simulink model "Automated_features1"  (R2020b)
settings: Solver=VariableStepAuto  StartTime=0.0  StopTime=10.0  RelTol=1e-3
undefined symbols (not defined in the file): sigbuilder_block
libraries: simulink x126
(part 1 of 3)
settings Model: Creator=99003762  LastModifiedBy=99003728
settings SFSimCC: CustomCodeUndefinedFunction=UseInterfaceOnly

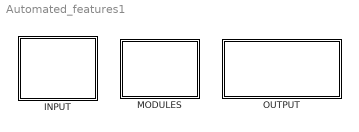
== system Automated_features1 ==
  INPUT : Subsystem
  MODULES : Subsystem
  OUTPUT : Subsystem

== system Automated_features1/INPUT ==
  note: Tier pressure sensors and Roof Control Inputs
  AIRBAG_INPUTS : Subsystem
  ALARM_INPUTS : Subsystem
  Cruise_Control_INPUT : Subsystem
  Power_window_ip : Subsystem  Tag=power_ip
  SEAT_RESTRAINT_INPUTS : Subsystem
  Signal Builder : Subsystem  Tag=STV Subsys  LoadFcn=sigbuilder_block('load');  StartFcn=sigbuilder_block('start');  StopFcn=sigbuilder_block('stop');  ClipboardFcn=sigbuilder_block('clipboard');  mask(Sigbuilder block){tuvar=[0:10]}
      mask help: Simulink:masks:SigbuilderBlock_MD
      mask init:
      | if ~strcmp(get_param(bdroot(gcbh),'SimulationStatus'),'stopped') tuvar = sigbuilder_block('maskInit'); end
      settings: CopyFcn=sigbuilder_block('copy');  DeleteFcn=sigbuilder_block('delete');  ModelCloseFcn=sigbuilder_block('modelClose');  PreSaveFcn=sigbuilder_block('preSave');  PauseFcn=sigbuilder_block('pause');  ContinueFcn=sigbuilder_block('continue');  NameChangeFcn=sigbuilder_block('namechange');  OpenFcn=sigbuilder_block('open',[6 30 1188 546.75 ]);  CloseFcn=sigbuilder_block('close');
      mask Display: plot(0, 0, 100, 100,[2, 2, 32, 32, 2], [68, 8, 8, 68, 68],[32, 2], [38, 38], [32, 19, 2],[53, 60, 44], [32, 17, 17, 2],[16, 16, 31, 31]);txt = getActiveGroup(gcbh);text(2, 100, txt,'verticalAlignment', 'top');
  Wiper_INPUTS : Subsystem
  tag scope: CL_SW=global, CL_VAL=global, OP_SW=global, OP_VAL=global, TP1_IP=global, TP2=global, TP3=global, TP4=global
  wires:
  Signal Builder/2(TP2) -> [TP2]
  Signal Builder/7(OPEN_VALUE) -> [OP_VAL]
  Signal Builder/1(TP1) -> [TP1_IP]
  Signal Builder/6(CLOSE_SW) -> [CL_SW]
  Signal Builder/4(TP4) -> [TP4]
  Signal Builder/3(TP3) -> [TP3]
  Signal Builder/5(OPEN_SW) -> [OP_SW]
  Signal Builder/8(CLOSE_VALUE) -> [CL_VAL]

== system Automated_features1/MODULES ==
  "\tPOWER_WINDOW" : Subsystem
  AIRBAGSYSTEM : Subsystem
  ALARM_SYSTEM : Subsystem
  CRUISE_CONTROL : Subsystem
  SeatBelt_MODULE : Subsystem
  Tire Pressure Monitoring System : Subsystem
  WIPER_CONTROL : Subsystem
  sunroof : Subsystem
  tag scope: CushionAngle=global, FrontAngle=global, RearAngle=global, SeatAdj=global
  wires:
  SeatBelt_MODULE/4(CushionAdjustAngle) -> [CushionAngle]
  SeatBelt_MODULE/2(RearAdjustAngle) -> [RearAngle]
  SeatBelt_MODULE/3(SeatAdjust) -> [SeatAdj]
  SeatBelt_MODULE/1(FrontAdjustAngle) -> [FrontAngle]

== system Automated_features1/OUTPUT ==
  note: sunroof Display
  note: Tyre pressure Indicators
  AIRBAG_OUTPUTS : Subsystem
  ALARM_OUTPUT1 : Subsystem
  Cruise_output : Subsystem
  OUTPUT1 : Subsystem
  OUTPUT2 : Subsystem
  Power_window_OUTPUT : Subsystem
  SeatBelt_OUTPUTS : Subsystem
  TP1_Indicator : LampBlock
  TP2_Indicator : LampBlock
  TP3_Indicator : LampBlock
  TP4_Indicator : LampBlock

== system Automated_features1/INPUT/AIRBAG_INPUTS ==
  Signal Builder : Subsystem  Tag=STV Subsys  LoadFcn=sigbuilder_block('load');  StartFcn=sigbuilder_block('start');  StopFcn=sigbuilder_block('stop');  ClipboardFcn=sigbuilder_block('clipboard');  mask(Sigbuilder block){tuvar=[0:10]}
      mask help: Simulink:masks:SigbuilderBlock_MD
      mask init:
      | if ~strcmp(get_param(bdroot(gcbh),'SimulationStatus'),'stopped') tuvar = sigbuilder_block('maskInit'); end
      settings: CopyFcn=sigbuilder_block('copy');  DeleteFcn=sigbuilder_block('delete');  ModelCloseFcn=sigbuilder_block('modelClose');  PreSaveFcn=sigbuilder_block('preSave');  PauseFcn=sigbuilder_block('pause');  ContinueFcn=sigbuilder_block('continue');  NameChangeFcn=sigbuilder_block('namechange');  OpenFcn=sigbuilder_block('open',[437.6 199.2 550.4 400 ]);  CloseFcn=sigbuilder_block('close');
      mask Display: plot(0, 0, 100, 100,[2, 2, 32, 32, 2], [68, 8, 8, 68, 68],[32, 2], [38, 38], [32, 19, 2],[53, 60, 44], [32, 17, 17, 2],[16, 16, 31, 31]);txt = getActiveGroup(gcbh);text(2, 100, txt,'verticalAlignment', 'top');
  tag scope: Air_ACC=global, Driver_L=global, L_Front_1=global, L_Rear_1=global, R_Rear_=global, VehicleSpeed=global, YawRate=global
  wires:
  Signal Builder/1(Driver_L) -> [Driver_L]
  Signal Builder/2(L_Front_1) -> [L_Front_1]
  Signal Builder/3(L_Rear_1) -> [L_Rear_1]
  Signal Builder/4(R_Rear_) -> [R_Rear_]
  Signal Builder/5(VehicleSpeed) -> [VehicleSpeed]
  Signal Builder/6(Air_ACC) -> [Air_ACC]
  Signal Builder/7(YawRate) -> [YawRate]

== system Automated_features1/INPUT/ALARM_INPUTS ==
  Signal Builder : Subsystem  Tag=STV Subsys  LoadFcn=sigbuilder_block('load');  StartFcn=sigbuilder_block('start');  StopFcn=sigbuilder_block('stop');  ClipboardFcn=sigbuilder_block('clipboard');  mask(Sigbuilder block){tuvar=[0:10]}
      mask help: Simulink:masks:SigbuilderBlock_MD
      mask init:
      | if ~strcmp(get_param(bdroot(gcbh),'SimulationStatus'),'stopped') tuvar = sigbuilder_block('maskInit'); end
      settings: CopyFcn=sigbuilder_block('copy');  DeleteFcn=sigbuilder_block('delete');  ModelCloseFcn=sigbuilder_block('modelClose');  PreSaveFcn=sigbuilder_block('preSave');  PauseFcn=sigbuilder_block('pause');  ContinueFcn=sigbuilder_block('continue');  NameChangeFcn=sigbuilder_block('namechange');  OpenFcn=sigbuilder_block('open',[403.5 199.2 550.5 359.55 ]);  CloseFcn=sigbuilder_block('close');
      mask Display: plot(0, 0, 100, 100,[2, 2, 32, 32, 2], [68, 8, 8, 68, 68],[32, 2], [38, 38], [32, 19, 2],[53, 60, 44], [32, 17, 17, 2],[16, 16, 31, 31]);txt = getActiveGroup(gcbh);text(2, 100, txt,'verticalAlignment', 'top');
  tag scope: AS_Doors=global, CAR_ON=global, Ignition=global, RKE=global
  wires:
  Signal Builder/1(AS_Doors) -> [AS_Doors]
  Signal Builder/2(Ignition) -> [Ignition]
  Signal Builder/3(Car_ON) -> [CAR_ON]
  Signal Builder/4(RKE) -> [RKE]

== system Automated_features1/INPUT/Cruise_Control_INPUT ==
  Signal Builder : Subsystem  Tag=STV Subsys  LoadFcn=sigbuilder_block('load');  StartFcn=sigbuilder_block('start');  StopFcn=sigbuilder_block('stop');  ClipboardFcn=sigbuilder_block('clipboard');  mask(Sigbuilder block){tuvar=[0:10]}
      mask help: Simulink:masks:SigbuilderBlock_MD
      mask init:
      | if ~strcmp(get_param(bdroot(gcbh),'SimulationStatus'),'stopped') tuvar = sigbuilder_block('maskInit'); end
      settings: CopyFcn=sigbuilder_block('copy');  DeleteFcn=sigbuilder_block('delete');  ModelCloseFcn=sigbuilder_block('modelClose');  PreSaveFcn=sigbuilder_block('preSave');  PauseFcn=sigbuilder_block('pause');  ContinueFcn=sigbuilder_block('continue');  NameChangeFcn=sigbuilder_block('namechange');  OpenFcn=sigbuilder_block('open',[437.6 153 550.4 359.25 ]);  CloseFcn=sigbuilder_block('close');
      mask Display: plot(0, 0, 100, 100,[2, 2, 32, 32, 2], [68, 8, 8, 68, 68],[32, 2], [38, 38], [32, 19, 2],[53, 60, 44], [32, 17, 17, 2],[16, 16, 31, 31]);txt = getActiveGroup(gcbh);text(2, 100, txt,'verticalAlignment', 'top');
  tag scope: BRAKE_CC=global, CRUISE_SPEED_CHANGE_SW=global, CRUISE_SWITCH=global, DESIRED_SPEED_CRUISE=global, ESC_cc=global, IGN=global, SPEED_CONTROL_CC=global, TSC_CC=global
  wires:
  Signal Builder/4(Ignition) -> [IGN]  "igswitch"
  Signal Builder/6(Cruise_switch) -> [CRUISE_SWITCH]
  Signal Builder/3(BRAKE) -> [BRAKE_CC]
  Signal Builder/5(desired_speed) -> [DESIRED_SPEED_CRUISE]
  Signal Builder/7(Speed_enable) -> [CRUISE_SPEED_CHANGE_SW]
  Signal Builder/2(TSC) -> [TSC_CC]
  Signal Builder/1(ESC) -> [ESC_cc]
  Signal Builder/8(Cruise_speed_change_sw) -> [SPEED_CONTROL_CC]

== system Automated_features1/INPUT/Power_window_ip ==
  Signal Builder : Subsystem  Tag=STV Subsys  LoadFcn=sigbuilder_block('load');  StartFcn=sigbuilder_block('start');  StopFcn=sigbuilder_block('stop');  ClipboardFcn=sigbuilder_block('clipboard');  mask(Sigbuilder block){tuvar=[0:10]}
      mask help: Simulink:masks:SigbuilderBlock_MD
      mask init:
      | if ~strcmp(get_param(bdroot(gcbh),'SimulationStatus'),'stopped') tuvar = sigbuilder_block('maskInit'); end
      settings: CopyFcn=sigbuilder_block('copy');  DeleteFcn=sigbuilder_block('delete');  ModelCloseFcn=sigbuilder_block('modelClose');  PreSaveFcn=sigbuilder_block('preSave');  PauseFcn=sigbuilder_block('pause');  ContinueFcn=sigbuilder_block('continue');  NameChangeFcn=sigbuilder_block('namechange');  OpenFcn=sigbuilder_block('open',[6 6 1012.5 506.25 ]);  CloseFcn=sigbuilder_block('close');
      mask Display: plot(0, 0, 100, 100,[2, 2, 32, 32, 2], [68, 8, 8, 68, 68],[32, 2], [38, 38], [32, 19, 2],[53, 60, 44], [32, 17, 17, 2],[16, 16, 31, 31]);txt = getActiveGroup(gcbh);text(2, 100, txt,'verticalAlignment', 'top');
  tag scope: Front_left_button_CP=global, Front_left_button_driver_side=global, driver_switch=global, ignition=global, lock_unlock_button=global, object=global, rear_left_button_CP=global, rear_left_button_driver_side=global, rear_right_button_CP=global, rear_right_button_driver_side=global
  wires:
  Signal Builder/5(Front_left_DC) -> [Front_left_button_driver_side]
  Signal Builder/9(Lock_Unlock) -> [lock_unlock_button]
  Signal Builder/6(rear_left_DC) -> [rear_left_button_driver_side]
  Signal Builder/8(oject_detection) -> [object]
  Signal Builder/3(Right_right_CP) -> [rear_right_button_CP]
  Signal Builder/7(rear_right_DC) -> [rear_right_button_driver_side]
  Signal Builder/2(Right_left_CP) -> [rear_left_button_CP]
  Signal Builder/1(Front_left_CP) -> [Front_left_button_CP]
  Signal Builder/10(iginition) -> [ignition]
  Signal Builder/4(Driver_control) -> [driver_switch]

== system Automated_features1/INPUT/SEAT_RESTRAINT_INPUTS ==
  tag scope: AdjustCushionAngle=global, AdjustFrontSeatAngle=global, AdjustRearSeatAngle=global, AdjustSeat=global, FrontSeat=global, HandleOn=global, ModeSelection=global, PowerSeat=global

== system Automated_features1/INPUT/Signal Builder ==
  Demux : Demux  Tag=STV Demux  Outputs=8
      settings: DisplayOption=none
  FromWs : FromWorkspace  Tag=STV FromWs  VariableName=tuvar  SampleTime=1
      SigBuilderData=|
      | common.afterFinalStr = 'Extrapolate'
      | common.sampleTime = '1'
      | dataSet.timeRange = [0 14]
      | dataSet.name = 'Sheet1'
      | sbobj.Name = 'Signal Builder'
      | sbobj.Groups.Name = 'Sheet1'
      | sbobj.Groups.Signals(1).Name = 'TP1'
      | sbobj.Groups.Signals(1).XData = [0 1 2 3 4 5 6 7 8 9 10 11 12 13 14]
      | sbobj.Groups.Signals(1).YData = [76 40 12 45 30 78 72 80 0 85 99 90 14 77 96]
      | sbobj.Groups.Signals(2).Name = 'TP2'
      | sbobj.Groups.Signals(2).XData = [0 1 2 3 4 5 6 7 8 9 10 11 12 13 14]
      | sbobj.Groups.Signals(2).YData = [76 40 96 45 30 78 72 80 0 85 99 90 14 77 96]
      | sbobj.Groups.Signals(3).Name = 'TP3'
      | sbobj.Groups.Signals(3).XData = [0 1 2 3 4 5 6 7 8 9 10 11 12 13 14]
      | sbobj.Groups.Signals(3).YData = [76 40 12 89 30 78 72 80 0 85 99 90 14 77 96]
      | sbobj.Groups.Signals(4).Name = 'TP4'
      | sbobj.Groups.Signals(4).XData = [0 1 2 3 4 5 6 7 8 9 10 11 12 13 14]
      | sbobj.Groups.Signals(4).YData = [76 80 82 45 1 78 72 80 0 85 99 90 14 77 96]
      | sbobj.Groups.Signals(5).Name = 'OPEN_SW'
      | sbobj.Groups.Signals(5).XData = [0 1 2 3 4 5 6 7 8 9 10 11 12 13 14]
      | sbobj.Groups.Signals(5).YData = [0 0 0 0 0 0 0 0 1 1 1 1 1 1 1]
      | sbobj.Groups.Signals(6).Name = 'CLOSE_SW'
      | sbobj.Groups.Signals(6).XData = [0 1 2 3 4 5 6 7 8 9 10 11 12 13 14]
      | sbobj.Groups.Signals(6).YData = [1 0 1 1 1 1 1 1 1 0 0 0 0 0 0]
      | sbobj.Groups.Signals(7).Name = 'OPEN_VALUE'
      | sbobj.Groups.Signals(7).XData = [0 1 2 3 4 5 6 7 8 9 10 11 12 13 14]
      | sbobj.Groups.Signals(7).YData = [76 40 12 45 30 78 72 80 0 85 99 90 14 77 96]
      | sbobj.Groups.Signals(8).Name = 'CLOSE_VALUE'
      | sbobj.Groups.Signals(8).XData = [0 1 2 3 4 5 6 7 8 9 10 11 12 13 14]
      | sbobj.Groups.Signals(8).YData = [76 40 12 45 30 78 72 80 0 85 99 90 14 77 96]
      | sbobj.Groups.TimeRange = [0 14]
  TP1 : Outport  Tag=STV Outport
  TP2 : Outport  Tag=STV Outport  Port=2
  TP3 : Outport  Tag=STV Outport  Port=3
  TP4 : Outport  Tag=STV Outport  Port=4
  OPEN_SW : Outport  Tag=STV Outport  Port=5
  CLOSE_SW : Outport  Tag=STV Outport  Port=6
  OPEN_VALUE : Outport  Tag=STV Outport  Port=7
  CLOSE_VALUE : Outport  Tag=STV Outport  Port=8
  wires:
  Demux/1 -> TP1/1
  FromWs/1 -> Demux/1
  Demux/2 -> TP2/1
  Demux/3 -> TP3/1
  Demux/4 -> TP4/1
  Demux/5 -> OPEN_SW/1
  Demux/6 -> CLOSE_SW/1
  Demux/7 -> OPEN_VALUE/1
  Demux/8 -> CLOSE_VALUE/1

== system Automated_features1/INPUT/Wiper_INPUTS ==
  Signal Builder : Subsystem  Tag=STV Subsys  LoadFcn=sigbuilder_block('load');  StartFcn=sigbuilder_block('start');  StopFcn=sigbuilder_block('stop');  ClipboardFcn=sigbuilder_block('clipboard');  mask(Sigbuilder block){tuvar=[0:10]}
      mask help: Simulink:masks:SigbuilderBlock_MD
      mask init:
      | if ~strcmp(get_param(bdroot(gcbh),'SimulationStatus'),'stopped') tuvar = sigbuilder_block('maskInit'); end
      settings: CopyFcn=sigbuilder_block('copy');  DeleteFcn=sigbuilder_block('delete');  ModelCloseFcn=sigbuilder_block('modelClose');  PreSaveFcn=sigbuilder_block('preSave');  PauseFcn=sigbuilder_block('pause');  ContinueFcn=sigbuilder_block('continue');  NameChangeFcn=sigbuilder_block('namechange');  OpenFcn=sigbuilder_block('open',[437.6 199.2 550.4 400 ]);  CloseFcn=sigbuilder_block('close');
      mask Display: plot(0, 0, 100, 100,[2, 2, 32, 32, 2], [68, 8, 8, 68, 68],[32, 2], [38, 38], [32, 19, 2],[53, 60, 44], [32, 17, 17, 2],[16, 16, 31, 31]);txt = getActiveGroup(gcbh);text(2, 100, txt,'verticalAlignment', 'top');
  tag scope: FC_ManualInput=global, FW_Modes=global, WC_BackS=global, WC_FrontS=global, WC_Status=global
  wires:
  Signal Builder/1(FC_Modes) -> [FW_Modes]
  Signal Builder/2(FC_ManualInput) -> [FC_ManualInput]
  Signal Builder/3(WC_BackS) -> [WC_BackS]
  Signal Builder/4(WC_Fronts) -> [WC_FrontS]
  Signal Builder/5(WC_Status) -> [WC_Status]

== system Automated_features1/MODULES/	POWER_WINDOW ==
  Subsystem4 : Subsystem
  tag scope: FL_out=global, FL_warn=global, RL_out=global, RL_warn=global, RR_out=global, RR_warn=global, driver_side_output=global, driver_warn=global
  wires:
  Subsystem4/2(Out_FL) -> [FL_out]
  Subsystem4/1(Out_warn) -> [FL_warn]
  Subsystem4/4(Out_RL) -> [RL_out]
  Subsystem4/6(Out_RR) -> [RR_out]
  [object] -> Subsystem4/2(object)
  [ignition] -> Subsystem4/1(Ig_sw)
  Subsystem4/3(Out_RL_warn) -> [RL_warn]
  Subsystem4/8(Out_DC) -> [driver_side_output]
  Subsystem4/5(Out_RR_warn) -> [RR_warn]
  Subsystem4/7(Out_DC_warn) -> [driver_warn]

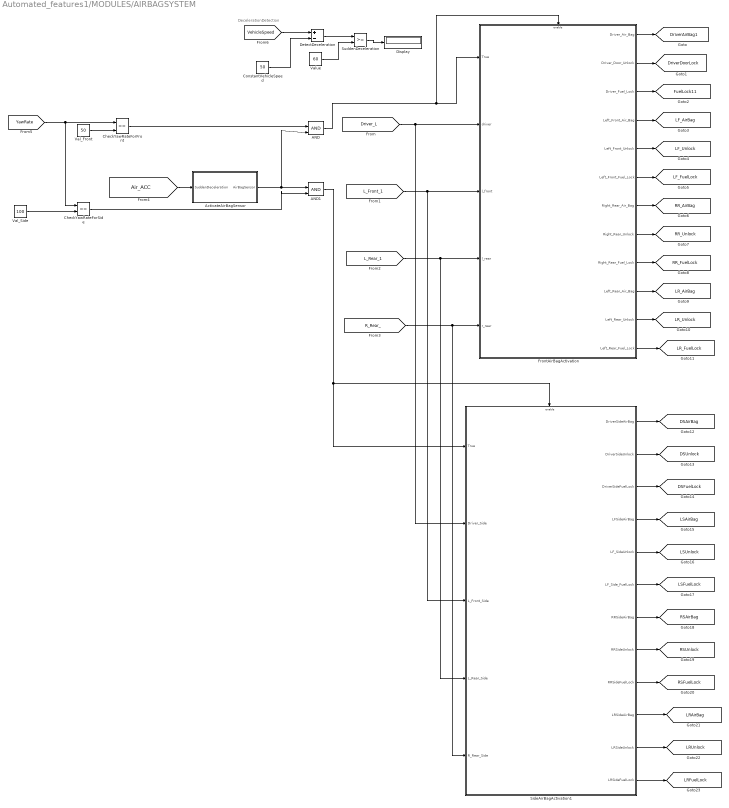
== system Automated_features1/MODULES/AIRBAGSYSTEM ==
  note: DecelerationDetection
  AND : Logic  IconShape=distinctive  AllPortsSameDT=off  OutDataTypeStr=boolean
  AND1 : Logic  IconShape=distinctive  AllPortsSameDT=off  OutDataTypeStr=boolean
  ActivateAirBagSensor : MATLAB Function  TreatAsAtomicUnit=on
  CheckYawRateForFront : RelationalOperator  Operator===  OutDataTypeStr=boolean  RndMeth=Simplest
  CheckYawRateForSide : RelationalOperator  Operator===  OutDataTypeStr=boolean  RndMeth=Simplest
  ConstantVehicleSpeed : Constant  Value=50
  DetectDeceleration : Sum  Inputs=+-
  Display : Display
  FrontAirBagActivation : Subsystem  TreatAsAtomicUnit=on
  SideAirBagActivation1 : Subsystem  TreatAsAtomicUnit=on
  SuddenDeceleration : RelationalOperator  OutDataTypeStr=boolean  RndMeth=Simplest
  Val_Front : Constant  Value=50
  Val_Side : Constant  Value=100
  Value : Constant  Value=60
  tag scope: DSAirBag=global, DSFuelLock=global, DSUnlock=global, DriverAirBag1=global, DriverDoorLock=global, FuelLock11=global, LF_AirBag=global, LF_FuelLock=global, LF_Unlock=global, LRAirBag=global, LRFuelLock=global, LRUnlock=global, LR_AirBag=global, LR_FuelLock=global, LR_Unlock=global, LSAirBag=global, LSFuelLock=global, LSUnlock=global, RR_AirBag=global, RR_FuelLock=global, RR_Unlock=global, RSAirBag=global, RSFuelLock=global, RSUnlock=global
  wires:
  CheckYawRateForFront/1 -> AND/1
  AND1/1 -> SideAirBagActivation1/1(True), SideAirBagActivation1/Enable
  ActivateAirBagSensor/1(AirBagSensor) -> AND1/1, AND/2
  [VehicleSpeed] -> DetectDeceleration/1
  ConstantVehicleSpeed/1 -> DetectDeceleration/2
  AND/1 -> FrontAirBagActivation/1(True), FrontAirBagActivation/Enable
  [Air_ACC] -> ActivateAirBagSensor/1(SuddenDeceleration)
  Value/1 -> SuddenDeceleration/2
  DetectDeceleration/1 -> SuddenDeceleration/1
  SuddenDeceleration/1 -> Display/1
  [YawRate] -> CheckYawRateForSide/1, CheckYawRateForFront/1
  Val_Side/1 -> CheckYawRateForSide/2
  [Driver_L] -> FrontAirBagActivation/2(driver), SideAirBagActivation1/2(Driver_Side)
  Val_Front/1 -> CheckYawRateForFront/2
  [R_Rear_] -> SideAirBagActivation1/5(R_Rear_Side), FrontAirBagActivation/5(r_rear)
  [L_Rear_1] -> SideAirBagActivation1/4(L_Rear_Side), FrontAirBagActivation/4(l_rear)
  [L_Front_1] -> FrontAirBagActivation/3(l_front), SideAirBagActivation1/3(L_Front_Side)
  CheckYawRateForSide/1 -> AND1/2
  FrontAirBagActivation/1(Driver_Air_Bag) -> [DriverAirBag1]
  FrontAirBagActivation/2(Driver_Door_Unlock) -> [DriverDoorLock]
  FrontAirBagActivation/3(Driver_Fuel_Lock) -> [FuelLock11]
  FrontAirBagActivation/4(Left_Front_Air_Bag) -> [LF_AirBag]
  FrontAirBagActivation/5(Left_Front_Unlock) -> [LF_Unlock]
  FrontAirBagActivation/6(Left_Front_Fuel_Lock) -> [LF_FuelLock]
  FrontAirBagActivation/7(Right_Rear_Air_Bag) -> [RR_AirBag]
  FrontAirBagActivation/8(Right_Rear_Unlock) -> [RR_Unlock]
  FrontAirBagActivation/9(Right_Rear_Fuel_Lock) -> [RR_FuelLock]
  FrontAirBagActivation/10(Left_Rear_Air_Bag) -> [LR_AirBag]
  FrontAirBagActivation/11(Left_Rear_Unlock) -> [LR_Unlock]
  FrontAirBagActivation/12(Left_Rear_Fuel_Lock) -> [LR_FuelLock]
  SideAirBagActivation1/1(DriverSideAirBag) -> [DSAirBag]
  SideAirBagActivation1/2(DriverSideUnlock) -> [DSUnlock]
  SideAirBagActivation1/3(DriverSideFuelLock) -> [DSFuelLock]
  SideAirBagActivation1/4(LFSideAirBag) -> [LSAirBag]
  SideAirBagActivation1/5(LF_SideUnlock) -> [LSUnlock]
  SideAirBagActivation1/6(LF_Side_FuelLock) -> [LSFuelLock]
  SideAirBagActivation1/7(RRSideAirBag) -> [RSAirBag]
  SideAirBagActivation1/8(RRSideUnlock) -> [RSUnlock]
  SideAirBagActivation1/9(RRSideFuelLock) -> [RSFuelLock]
  SideAirBagActivation1/10(LRSideAirBag) -> [LRAirBag]
  SideAirBagActivation1/11(LRSideUnlock) -> [LRUnlock]
  SideAirBagActivation1/12(LRSideFuelLock) -> [LRFuelLock]

== system Automated_features1/MODULES/ALARM_SYSTEM ==
  AND : Logic  Inputs=3  IconShape=distinctive  AllPortsSameDT=off  OutDataTypeStr=boolean
  AND1 : Logic  Inputs=3  IconShape=distinctive  AllPortsSameDT=off  OutDataTypeStr=boolean
  AND2 : Logic  IconShape=distinctive  AllPortsSameDT=off  OutDataTypeStr=boolean
  AND3 : Logic  IconShape=distinctive  AllPortsSameDT=off  OutDataTypeStr=boolean
  ARMED : Stateflow chart  TreatAsAtomicUnit=on
  Compare To Constant : simulink/Logic and Bit Operations/Compare To Constant  relop===  const=0  OutDataTypeStr=boolean
  Compare To Constant2 : simulink/Logic and Bit Operations/Compare To Constant  relop===  const=1  OutDataTypeStr=boolean
  Compare To Constant3 : simulink/Logic and Bit Operations/Compare To Constant  relop===  const=1  OutDataTypeStr=boolean
  Compare To Zero : simulink/Logic and Bit Operations/Compare To Zero  relop===  OutDataTypeStr=boolean
  Compare To Zero1 : simulink/Logic and Bit Operations/Compare To Zero  relop===  OutDataTypeStr=boolean
  Constant : Constant
  Constant1 : Constant
  Constant2 : Constant
  Constant3 : Constant  Value=0
  Display : Display
  Main_Alarm : Subsystem  Commented=on
  NAND : Logic  Operator=NAND  IconShape=distinctive  AllPortsSameDT=off  OutDataTypeStr=boolean
  Pre_Alarm : Stateflow chart  TreatAsAtomicUnit=on
  Slider Switch : SliderSwitchBlock  Commented=on
      settings: Values={{'Off', 'On'}, [1 0]}
  Switch : Switch  Criteria=u2 ~= 0
  Switch1 : Switch  Criteria=u2 ~= 0
  Switch2 : Switch  Criteria=u2 ~= 0
  tag scope: Alarm_ARMED=global, Disarmed=global, Prealarm_ARMED=global
  wires:
  [RKE] -> AND1/2, Compare To Zero/1, AND2/2  "RKE"
  Constant/1 -> Switch/1
  Constant1/1 -> Switch1/1
  Compare To Zero1/1 -> AND3/2
  Compare To Constant3/1 -> NAND/1
  [CAR_ON] -> AND/2
  Compare To Zero/1 -> AND3/1
  AND2/1 -> ARMED/1(data)
  Pre_Alarm/1(data1) -> Switch1/2
  Compare To Constant/1 -> AND2/1
  AND1/1 -> Switch/2
  [Ignition] -> Compare To Constant2/1, AND/1
  AND/1 -> Compare To Constant/1
  Compare To Constant2/1 -> AND1/1
  Switch/1 -> Switch2/2, [Disarmed]
  Switch1/1 -> [Prealarm_ARMED]
  ARMED/1(data1) -> AND1/3, Compare To Constant3/1
  AND3/1 -> Pre_Alarm/1(data)
  [AS_Doors] -> Display/1, Compare To Zero1/1, AND/3
  Constant2/1 -> Switch2/1
  Switch2/1 -> NAND/2
  NAND/1 -> [Alarm_ARMED]
  Constant3/1 -> Switch2/3

== system Automated_features1/MODULES/CRUISE_CONTROL ==
  note: IGN
  Display : Display
  MATLAB Function : MATLAB Function  TreatAsAtomicUnit=on
  tag scope: output_cruise=global
  wires:
  [DESIRED_SPEED_CRUISE] -> MATLAB Function/5(DESIRED_SPEED_CRUISE)
  [BRAKE_CC] -> MATLAB Function/3(BRAKE_CC)
  [CRUISE_SWITCH] -> MATLAB Function/6(cs)
  [ESC_cc] -> MATLAB Function/1(ESC_CC)
  [SPEED_CONTROL_CC] -> MATLAB Function/8(speedch)
  MATLAB Function/1(y) -> [output_cruise], Display/1  "output"
  [TSC_CC] -> MATLAB Function/2(TSC_CC)
  [IGN] -> MATLAB Function/4(IGN)
  [CRUISE_SPEED_CHANGE_SW] -> MATLAB Function/7(CRUISE_SPEED_CHANGE_SW)

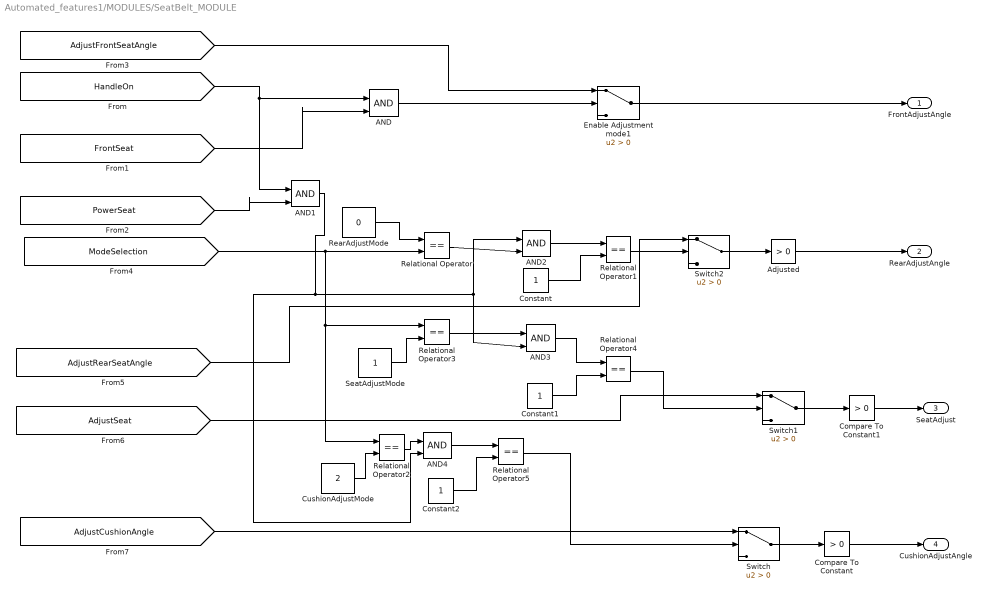
== system Automated_features1/MODULES/SeatBelt_MODULE ==
  AND{,1..4} (5 alike) : Logic  IconShape=distinctive  AllPortsSameDT=off  OutDataTypeStr=boolean
  Adjusted : simulink/Logic and Bit Operations/Compare To Constant  relop=>  const=0  OutDataTypeStr=boolean
  Compare To Constant : simulink/Logic and Bit Operations/Compare To Constant  relop=>  const=0  OutDataTypeStr=boolean
  Compare To Constant1 : simulink/Logic and Bit Operations/Compare To Constant  relop=>  const=0  OutDataTypeStr=boolean
  Constant : Constant
  Constant1 : Constant
  Constant2 : Constant
  CushionAdjustMode : Constant  Value=2
  Enable Adjustment mode1 : Switch  Criteria=u2 > Threshold
  RearAdjustMode : Constant  Value=0
  Relational Operator{,1..5} (6 alike) : RelationalOperator  Operator===  OutDataTypeStr=boolean  RndMeth=Simplest
  SeatAdjustMode : Constant
  Switch : Switch  Criteria=u2 > Threshold
  Switch1 : Switch  Criteria=u2 > Threshold
  Switch2 : Switch  Criteria=u2 > Threshold
  FrontAdjustAngle : Outport
  RearAdjustAngle : Outport  Port=2
  SeatAdjust : Outport  Port=3
  CushionAdjustAngle : Outport  Port=4
  wires:
  AND3/1 -> Relational Operator4/1
  Compare To Constant/1 -> CushionAdjustAngle/1
  AND1/1 -> AND4/2, AND2/1, AND3/2
  [HandleOn] -> AND1/1, AND/1
  Switch2/1 -> Adjusted/1
  RearAdjustMode/1 -> Relational Operator/1
  [AdjustCushionAngle] -> Switch/1
  AND2/1 -> Relational Operator1/1
  AND/1 -> Enable Adjustment mode1/2
  Relational Operator2/1 -> AND4/1
  Compare To Constant1/1 -> SeatAdjust/1
  Constant/1 -> Relational Operator1/2
  [AdjustSeat] -> Switch1/1
  Relational Operator4/1 -> Switch1/2
  Switch/1 -> Compare To Constant/1
  Switch1/1 -> Compare To Constant1/1
  Relational Operator/1 -> AND2/2
  [FrontSeat] -> AND/2
  [AdjustRearSeatAngle] -> Switch2/1
  [ModeSelection] -> Relational Operator/2, Relational Operator2/1, Relational Operator3/1
  AND4/1 -> Relational Operator5/1
  Relational Operator3/1 -> AND3/1
  SeatAdjustMode/1 -> Relational Operator3/2
  Constant2/1 -> Relational Operator5/2
  Constant1/1 -> Relational Operator4/2
  [AdjustFrontSeatAngle] -> Enable Adjustment mode1/1
  Relational Operator1/1 -> Switch2/2
  Relational Operator5/1 -> Switch/2
  CushionAdjustMode/1 -> Relational Operator2/2
  [PowerSeat] -> AND1/2
  Adjusted/1 -> RearAdjustAngle/1
  Enable Adjustment mode1/1 -> FrontAdjustAngle/1

== system Automated_features1/MODULES/Tire Pressure Monitoring System ==
  TP_Monitoring : Subsystem
  Tier1State : Display
  Tier2State : Display
  Tier3State : Display
  Tier4State : Display
  wires:
  TP_Monitoring/2(Out2) -> Tier2State/1
  [TP4] -> TP_Monitoring/4(tierPressure4a), TP_Monitoring/8(tierPressure4b)
  TP_Monitoring/1(Out1) -> Tier1State/1
  [TP1_IP] -> TP_Monitoring/1(tierPressure1a), TP_Monitoring/5(tierPressure1b)
  [TP3] -> TP_Monitoring/7(tierPressure3b), TP_Monitoring/3(tierPressure3a)
  TP_Monitoring/3(Out3) -> Tier3State/1
  [TP2] -> TP_Monitoring/6(tierPressure2b), TP_Monitoring/2(tierPressure2a)
  TP_Monitoring/4(Out4) -> Tier4State/1

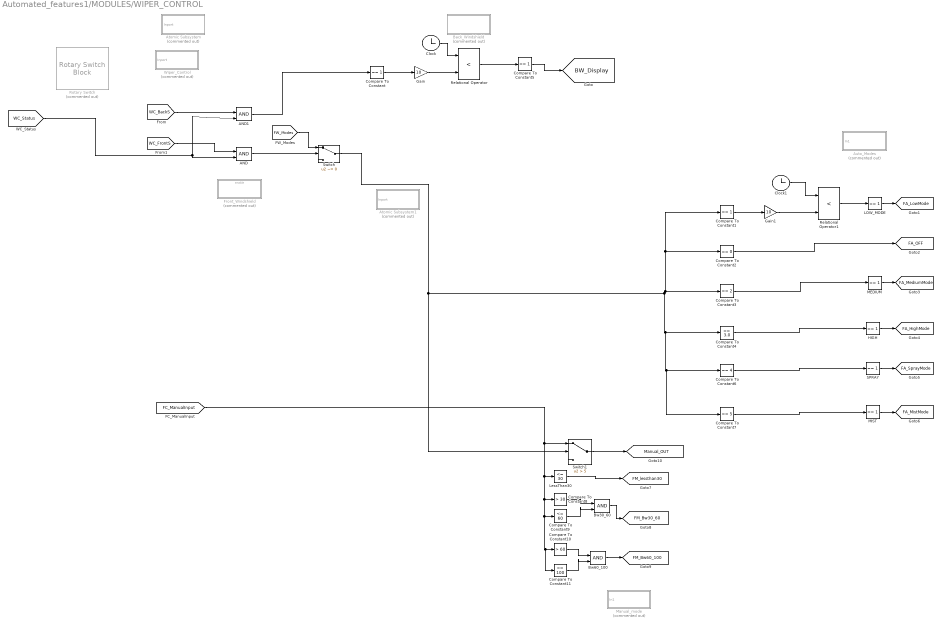
== system Automated_features1/MODULES/WIPER_CONTROL ==
  AND : Logic  IconShape=distinctive  AllPortsSameDT=off  OutDataTypeStr=boolean
  AND1 : Logic  IconShape=distinctive  AllPortsSameDT=off  OutDataTypeStr=boolean
  Atomic Subsystem : Subsystem  Commented=on  TreatAsAtomicUnit=on
  Atomic Subsystem1 : Subsystem  Commented=on  TreatAsAtomicUnit=on
  Auto_Modes : Subsystem  Commented=on
  Back_Windshield : Subsystem  Commented=on  TreatAsAtomicUnit=on
  Bw30_60 : Logic  IconShape=distinctive  AllPortsSameDT=off  OutDataTypeStr=boolean
  Bw60_100 : Logic  IconShape=distinctive  AllPortsSameDT=off  OutDataTypeStr=boolean
  Clock : Clock
      settings: Decimation=5
  Clock1 : Clock
      settings: Decimation=5
  Compare To Constant : simulink/Logic and Bit Operations/Compare To Constant  relop===  const=1  OutDataTypeStr=boolean
  Compare To Constant1 : simulink/Logic and Bit Operations/Compare To Constant  relop===  const=1  OutDataTypeStr=boolean
  Compare To Constant10 : simulink/Logic and Bit Operations/Compare To Constant  relop=>  const=60  OutDataTypeStr=boolean
  Compare To Constant11 : simulink/Logic and Bit Operations/Compare To Constant  relop=<=  const=100  OutDataTypeStr=boolean
  Compare To Constant2 : simulink/Logic and Bit Operations/Compare To Constant  relop===  const=0  OutDataTypeStr=boolean
  Compare To Constant3 : simulink/Logic and Bit Operations/Compare To Constant  relop===  const=2  OutDataTypeStr=boolean
  Compare To Constant4 : simulink/Logic and Bit Operations/Compare To Constant  relop===  const=3.0  OutDataTypeStr=boolean
  Compare To Constant5 : simulink/Logic and Bit Operations/Compare To Constant  relop===  const=1  OutDataTypeStr=boolean
  Compare To Constant6 : simulink/Logic and Bit Operations/Compare To Constant  relop===  const=4  OutDataTypeStr=boolean
  Compare To Constant7 : simulink/Logic and Bit Operations/Compare To Constant  relop===  const=5  OutDataTypeStr=boolean
  Compare To Constant8 : simulink/Logic and Bit Operations/Compare To Constant  relop=>  const=30  OutDataTypeStr=boolean
  Compare To Constant9 : simulink/Logic and Bit Operations/Compare To Constant  relop=<=  const=60  OutDataTypeStr=boolean
  Front_Windshield : Subsystem  Commented=on  TreatAsAtomicUnit=on
  Gain : Gain  Gain=10
  Gain1 : Gain  Gain=10
  HIGH : simulink/Logic and Bit Operations/Compare To Constant  relop===  const=1  OutDataTypeStr=boolean
  LOW_MODE : simulink/Logic and Bit Operations/Compare To Constant  relop===  const=1  OutDataTypeStr=boolean
  LessThan30 : simulink/Logic and Bit Operations/Compare To Constant  relop=<=  const=30  OutDataTypeStr=boolean
  MEDIUM : simulink/Logic and Bit Operations/Compare To Constant  relop===  const=1  OutDataTypeStr=boolean
  MIST : simulink/Logic and Bit Operations/Compare To Constant  relop===  const=1  OutDataTypeStr=boolean
  Manual_mode : Subsystem  Commented=on
  Relational Operator : RelationalOperator  Operator=<  OutDataTypeStr=boolean  RndMeth=Simplest
  Relational Operator1 : RelationalOperator  Operator=<  OutDataTypeStr=boolean  RndMeth=Simplest
  Rotary Switch : RotarySwitchBlock  Commented=on
      settings: Values={{'Off', 'Accessory', 'Ignition'}, [0 1 2]}
  SPRAY : simulink/Logic and Bit Operations/Compare To Constant  relop===  const=1  OutDataTypeStr=boolean
  Switch : Switch  Criteria=u2 ~= 0
  Switch1 : Switch  Criteria=u2 > Threshold  Threshold=5
  Wiper_Control : Subsystem  Commented=on  TreatAsAtomicUnit=on
  tag scope: BW_Display=global, FA_HighMode=global, FA_LowMode=global, FA_MediumMode=global, FA_MistMode=global, FA_OFF=global, FA_SprayMode=global, FM_Bw30_60=global, FM_Bw60_100=global, FM_lessthan30=global, Manual_OUT=global
  wires:
  [WC_Status] -> AND1/2, AND/2
  [WC_BackS] -> AND1/1
  [WC_FrontS] -> AND/1
  Compare To Constant/1 -> Gain/1
  Relational Operator/1 -> Compare To Constant5/1
  Compare To Constant5/1 -> [BW_Display]
  Gain/1 -> Relational Operator/2
  Clock/1 -> Relational Operator/1
  AND1/1 -> Compare To Constant/1
  AND/1 -> Switch/2
  [FW_Modes] -> Switch/1
  Compare To Constant6/1 -> SPRAY/1
  MEDIUM/1 -> [FA_MediumMode]
  HIGH/1 -> [FA_HighMode]
  LOW_MODE/1 -> [FA_LowMode]
  Relational Operator1/1 -> LOW_MODE/1
  Clock1/1 -> Relational Operator1/1
  Gain1/1 -> Relational Operator1/2
  SPRAY/1 -> [FA_SprayMode]
  MIST/1 -> [FA_MistMode]
  Compare To Constant7/1 -> MIST/1
  Compare To Constant2/1 -> [FA_OFF]
  Compare To Constant1/1 -> Gain1/1
  Switch1/1 -> [Manual_OUT]
  [FC_ManualInput] -> Compare To Constant11/1, Compare To Constant10/1, Compare To Constant9/1, Compare To Constant8/1, LessThan30/1, Switch1/1
  Compare To Constant9/1 -> Bw30_60/2
  Switch/1 -> Switch1/2, Compare To Constant7/1, Compare To Constant6/1, Compare To Constant4/1, Compare To Constant3/1, Compare To Constant1/1, Compare To Constant2/1
  LessThan30/1 -> [FM_lessthan30]
  Compare To Constant10/1 -> Bw60_100/1
  Compare To Constant8/1 -> Bw30_60/1
  Compare To Constant11/1 -> Bw60_100/2
  Bw60_100/1 -> [FM_Bw60_100]
  Bw30_60/1 -> [FM_Bw30_60]
  Compare To Constant3/1 -> MEDIUM/1
  Compare To Constant4/1 -> HIGH/1

== system Automated_features1/MODULES/sunroof ==
  Subsystem : Subsystem
  Subsystem1 : Subsystem
  enabling system : Subsystem
  tag scope: output1=global, output2=global
  wires:
  enabling system/1(Outport) -> Subsystem1/1(Enable)
  enabling system/2(enableO) -> Subsystem/1(Enable)
  [CL_VAL] -> Subsystem/2(Inport)
  [OP_VAL] -> Subsystem1/2(Inport)
  Subsystem/1(Outport) -> [output2]
  Subsystem1/1(Outport) -> [output1]

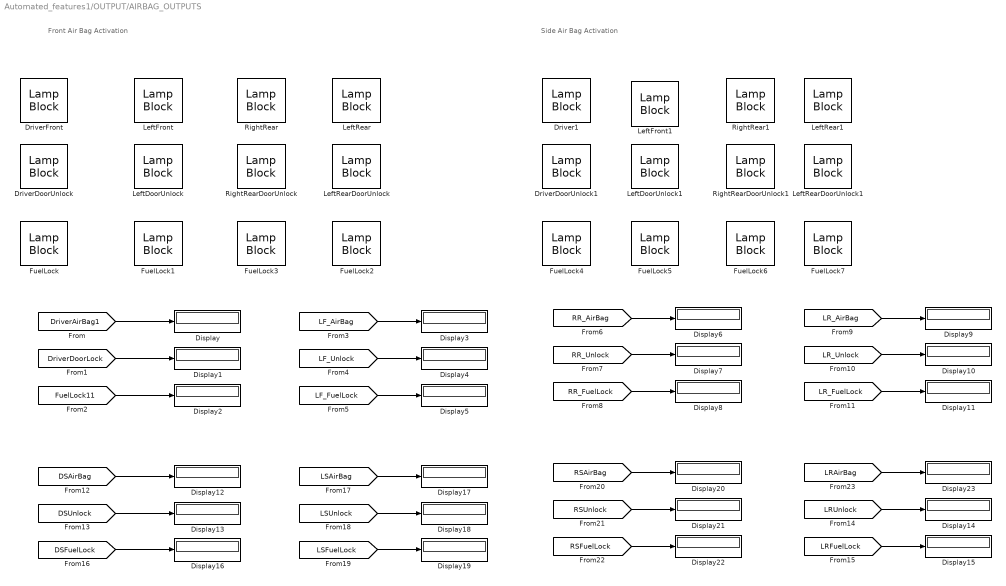
== system Automated_features1/OUTPUT/AIRBAG_OUTPUTS ==
  note: Front Air Bag Activation
  note: Side Air Bag Activation
  Display{,1..23} (24 alike) : Display
  Driver1 : LampBlock
  DriverDoorUnlock : LampBlock
  DriverDoorUnlock1 : LampBlock
  DriverFront : LampBlock
  FuelLock{,1..7} (8 alike) : LampBlock
  LeftDoorUnlock : LampBlock
  LeftDoorUnlock1 : LampBlock
  LeftFront : LampBlock
  LeftFront1 : LampBlock
  LeftRear : LampBlock
  LeftRear1 : LampBlock
  LeftRearDoorUnlock : LampBlock
  LeftRearDoorUnlock1 : LampBlock
  RightRear : LampBlock
  RightRear1 : LampBlock
  RightRearDoorUnlock : LampBlock
  RightRearDoorUnlock1 : LampBlock
  wires:
  [DriverAirBag1] -> Display/1
  [DriverDoorLock] -> Display1/1
  [FuelLock11] -> Display2/1
  [LF_AirBag] -> Display3/1
  [LF_Unlock] -> Display4/1
  [LF_FuelLock] -> Display5/1
  [RR_AirBag] -> Display6/1
  [RR_Unlock] -> Display7/1
  [RR_FuelLock] -> Display8/1
  [LR_AirBag] -> Display9/1
  [LR_Unlock] -> Display10/1
  [LR_FuelLock] -> Display11/1
  [DSFuelLock] -> Display16/1
  [LRAirBag] -> Display23/1
  [RSUnlock] -> Display21/1
  [RSAirBag] -> Display20/1
  [RSFuelLock] -> Display22/1
  [DSUnlock] -> Display13/1
  [LSUnlock] -> Display18/1
  [LRUnlock] -> Display14/1
  [LSFuelLock] -> Display19/1
  [LSAirBag] -> Display17/1
  [LRFuelLock] -> Display15/1
  [DSAirBag] -> Display12/1

== system Automated_features1/OUTPUT/ALARM_OUTPUT1 ==
  note: OUTPUTS
  Display : Display
  Display1 : Display
  Display2 : Display
  Lamp : LampBlock
  wires:
  [Disarmed] -> Display2/1
  [Prealarm_ARMED] -> Display1/1
  [Alarm_ARMED] -> Display/1

== system Automated_features1/OUTPUT/Cruise_output ==
  Gauge : CircularGaugeBlock
  Scope : Scope
  wires:
  [output_cruise] -> Scope/1

== system Automated_features1/OUTPUT/OUTPUT1 ==
  Display : Display
  Display1 : Display
  wires:
  [output2] -> Display1/1
  [output1] -> Display/1

== system Automated_features1/OUTPUT/OUTPUT2 ==
  note: BACK WINDSHIELD
  note: FRONT WINDSHIELD AUTOMODES
  note: FRONT WINDSHIELD MANUAL MANUAL OUTPUT
  Display{,1..10} (11 alike) : Display
  Lamp{,1..8} (9 alike) : LampBlock
  wires:
  [BW_Display] -> Display/1
  [FM_lessthan30] -> Display1/1
  [FM_Bw30_60] -> Display2/1
  [FM_Bw60_100] -> Display3/1
  [FA_LowMode] -> Display4/1
  [FA_MediumMode] -> Display5/1
  [FA_HighMode] -> Display6/1
  [FA_MistMode] -> Display7/1
  [FA_OFF] -> Display8/1
  [FA_SprayMode] -> Display9/1
  [Manual_OUT] -> Display10/1

== system Automated_features1/OUTPUT/Power_window_OUTPUT ==
  Output_window_scope : Scope  NumInputPorts=4
  Warning_Scope : Scope  NumInputPorts=4
  wires:
  [RR_warn] -> Warning_Scope/3
  [RL_warn] -> Warning_Scope/2
  [FL_warn] -> Warning_Scope/1
  [FL_out] -> Output_window_scope/1
  [RL_out] -> Output_window_scope/2
  [RR_out] -> Output_window_scope/3
  [driver_side_output] -> Output_window_scope/4
  [driver_warn] -> Warning_Scope/4

== system Automated_features1/OUTPUT/SeatBelt_OUTPUTS ==
  Display{,1..3} (4 alike) : Display
  wires:
  [RearAngle] -> Display1/1
  [SeatAdj] -> Display2/1
  [FrontAngle] -> Display/1
  [CushionAngle] -> Display3/1

== system Automated_features1/INPUT/AIRBAG_INPUTS/Signal Builder ==
  Demux : Demux  Tag=STV Demux  Outputs=7
      settings: DisplayOption=none
  FromWs : FromWorkspace  Tag=STV FromWs  VariableName=tuvar
      SigBuilderData=|
      | common.afterFinalStr = 'Extrapolate'
      | common.sampleTime = 0
      | dataSet.timeRange = [0 10]
      | dataSet.name = 'Group 1'
      | sbobj.Groups.Name = 'Group 1'
      | sbobj.Groups.Signals(1).Name = 'Driver_L'
      | sbobj.Groups.Signals(1).XData = [0 1 2 3 4 5 6 7 10]
      | sbobj.Groups.Signals(1).YData = [0 1 1 1 1 1 1 0 0]
      | sbobj.Groups.Signals(2).Name = 'L_Front_1'
      | sbobj.Groups.Signals(2).XData = [0 1 2 3 4 5 6 7 10]
      | sbobj.Groups.Signals(2).YData = [0 0 0 0 0 0 0 0 0]
      | sbobj.Groups.Signals(3).Name = 'L_Rear_1'
      | sbobj.Groups.Signals(3).XData = [0 1 2 3 4 5 6 7 10]
      | sbobj.Groups.Signals(3).YData = [0 0 0 0 0 0 0 0 0]
      | sbobj.Groups.Signals(4).Name = 'R_Rear_'
      | sbobj.Groups.Signals(4).XData = [0 1 2 3 4 5 6 7 10]
      | sbobj.Groups.Signals(4).YData = [0 0 0 0 0 0 0 1 1]
      | sbobj.Groups.Signals(5).Name = 'VehicleSpeed'
      | sbobj.Groups.Signals(5).XData = [0 1 2 3 4 5 6 7 10]
      | sbobj.Groups.Signals(5).YData = [0 50 50 140 140 140 140 140 140]
      | sbobj.Groups.Signals(6).Name = 'Air_ACC'
      | sbobj.Groups.Signals(6).XData = [0 1 2 3 4 5 6 7 10]
      | sbobj.Groups.Signals(6).YData = [0 0 0 1 1 1 1 1 1]
      | sbobj.Groups.Signals(7).Name = 'YawRate'
      | sbobj.Groups.Signals(7).XData = [0 1 2 3 4 5 6 7 8 10]
      | sbobj.Groups.Signals(7).YData = [0 50 50 50 50 100 100 50 100 100]
  Driver_L : Outport  Tag=STV Outport
  L_Front_1 : Outport  Tag=STV Outport  Port=2
  L_Rear_1 : Outport  Tag=STV Outport  Port=3
  R_Rear_ : Outport  Tag=STV Outport  Port=4
  VehicleSpeed : Outport  Tag=STV Outport  Port=5
  Air_ACC : Outport  Tag=STV Outport  Port=6
  YawRate : Outport  Tag=STV Outport  Port=7
  wires:
  FromWs/1 -> Demux/1
  Demux/1 -> Driver_L/1
  Demux/2 -> L_Front_1/1
  Demux/3 -> L_Rear_1/1
  Demux/4 -> R_Rear_/1
  Demux/5 -> VehicleSpeed/1
  Demux/6 -> Air_ACC/1
  Demux/7 -> YawRate/1

== system Automated_features1/INPUT/ALARM_INPUTS/Signal Builder ==
  Demux : Demux  Tag=STV Demux
      settings: DisplayOption=none
  FromWs : FromWorkspace  Tag=STV FromWs  VariableName=tuvar
      SigBuilderData=|
      | common.afterFinalStr = 'Extrapolate'
      | common.sampleTime = 0
      | dataSet.timeRange = [0 12]
      | dataSet.name = 'Group 1'
      | sbobj.Groups.Name = 'Group 1'
      | sbobj.Groups.Signals(1).Name = 'AS_Doors'
      | sbobj.Groups.Signals(1).XData = [0 1 2 3 4 5 6 7 8 9 10 11 12]
      | sbobj.Groups.Signals(1).YData = [0 1 1 1 1 1 1 1 1 1 1 1 1]
      | sbobj.Groups.Signals(2).Name = 'Ignition'
      | sbobj.Groups.Signals(2).XData = [0 1 2 3 4 5 6 7 8 9 10 11 12]
      | sbobj.Groups.Signals(2).YData = [0 1 1 1 1 1 1 1 1 1 1 1 1]
      | sbobj.Groups.Signals(3).Name = 'Car_ON'
      | sbobj.Groups.Signals(3).XData = [0 1 2 3 4 5 6 7 8 9 10 11 12]
      | sbobj.Groups.Signals(3).YData = [0 1 1 1 1 1 1 1 1 1 1 1 1]
      | sbobj.Groups.Signals(4).Name = 'RKE'
      | sbobj.Groups.Signals(4).XData = [0 1 2 3 4 5 6 7 8 9 10 11 12]
      | sbobj.Groups.Signals(4).YData = [0 1 1 1 1 1 2 2 2 2 2 2 2]
      | sbobj.Groups.TimeRange = [0 12]
  AS_Doors : Outport  Tag=STV Outport
  Ignition : Outport  Tag=STV Outport  Port=2
  Car_ON : Outport  Tag=STV Outport  Port=3
  RKE : Outport  Tag=STV Outport  Port=4
  wires:
  FromWs/1 -> Demux/1
  Demux/1 -> AS_Doors/1
  Demux/2 -> Ignition/1
  Demux/3 -> Car_ON/1
  Demux/4 -> RKE/1

== system Automated_features1/INPUT/Cruise_Control_INPUT/Signal Builder ==
  Demux : Demux  Tag=STV Demux  Outputs=8
      settings: DisplayOption=none
  FromWs : FromWorkspace  Tag=STV FromWs  VariableName=tuvar  SampleTime=1
      SigBuilderData=|
      | common.afterFinalStr = 'Extrapolate'
      | common.sampleTime = '1'
      | dataSet.timeRange = [0 20]
      | dataSet.name = 'Sheet1'
      | sbobj.Name = 'Signal Builder'
      | sbobj.Groups.Name = 'Sheet1'
      | sbobj.Groups.Signals(1).Name = 'ESC'
      | sbobj.Groups.Signals(1).XData = [0 1 2 3 4 5 6 7 8 9 10 11 12 13 14 15 16 17 18 19 20]
      | sbobj.Groups.Signals(1).YData = [1 0 0 0 0 0 0 0 0 0 0 0 0 0 0 0 0 0 0 0 0]
      | sbobj.Groups.Signals(2).Name = 'TSC'
      | sbobj.Groups.Signals(2).XData = [0 1 2 3 4 5 6 7 8 9 10 11 12 13 14 15 16 17 18 19 20]
      | sbobj.Groups.Signals(2).YData = [0 1 0 0 0 0 0 0 0 0 0 0 0 0 0 0 0 0 0 0 0]
      | sbobj.Groups.Signals(3).Name = 'BRAKE'
      | sbobj.Groups.Signals(3).XData = [0 1 2 3 4 5 6 7 8 9 10 11 12 13 14 15 16 17 18 19 20]
      | sbobj.Groups.Signals(3).YData = [0 1 1 0 0 0 0 0 0 0 0 0 0 0 0 0 0 0 0 0 0]
      | sbobj.Groups.Signals(4).Name = 'Ignition'
      | sbobj.Groups.Signals(4).XData = [0 1 2 3 4 5 6 7 8 9 10 11 12 13 14 15 16 17 18 19 20]
      | sbobj.Groups.Signals(4).YData = [1 0 0 0 1 1 1 1 1 1 1 1 1 1 1 1 1 1 1 1 1]
      | sbobj.Groups.Signals(5).Name = 'desired_speed'
      | sbobj.Groups.Signals(5).XData = [0 1 2 3 4 5 6 7 8 9 10 11 12 13 14 15 16 17 18 19 20]
      | sbobj.Groups.Signals(5).YData = [40.5 55 60 12 50 40 32.2 78 12 44 59 39 41 42 46 80 35 70 15 46 25]
      | sbobj.Groups.Signals(6).Name = 'Cruise_switch'
      | sbobj.Groups.Signals(6).XData = [0 1 2 3 4 5 6 7 8 9 10 11 12 13 14 15 16 17 18 19 20]
      | sbobj.Groups.Signals(6).YData = [0 0 0 0 0 0 1 1 1 0 1 0 1 0 1 1 1 1 1 1 1]
      | sbobj.Groups.Signals(7).Name = 'Speed_enable'
      | sbobj.Groups.Signals(7).XData = [0 1 2 3 4 5 6 7 8 9 10 11 12 13 14 15 16 17 18 19 20]
      | sbobj.Groups.Signals(7).YData = [1 1 1 0 0 1 1 1 0 1 1 0 1 1 0 1 1 1 0 1 0]
      | sbobj.Groups.Signals(8).Name = 'Cruise_speed_change_sw'
      | sbobj.Groups.Signals(8).XData = [0 1 2 3 4 5 6 7 8 9 10 11 12 13 14 15 16 17 18 19 20]
      | sbobj.Groups.Signals(8).YData = [10 20 12 10 5 20 17 13 14 25 15 19 23 20 5 10 12 3 30 0 15]
      | sbobj.Groups.TimeRange = [0 20]
  ESC : Outport  Tag=STV Outport
  TSC : Outport  Tag=STV Outport  Port=2
  BRAKE : Outport  Tag=STV Outport  Port=3
  Ignition : Outport  Tag=STV Outport  Port=4
  desired_speed : Outport  Tag=STV Outport  Port=5
  Cruise_switch : Outport  Tag=STV Outport  Port=6
  Speed_enable : Outport  Tag=STV Outport  Port=7
  Cruise_speed_change_sw : Outport  Tag=STV Outport  Port=8
  wires:
  Demux/1 -> ESC/1
  FromWs/1 -> Demux/1
  Demux/2 -> TSC/1
  Demux/3 -> BRAKE/1
  Demux/4 -> Ignition/1
  Demux/5 -> desired_speed/1
  Demux/6 -> Cruise_switch/1
  Demux/7 -> Speed_enable/1
  Demux/8 -> Cruise_speed_change_sw/1

== system Automated_features1/INPUT/Power_window_ip/Signal Builder ==
  Demux : Demux  Tag=STV Demux  Outputs=10
      settings: DisplayOption=none
  FromWs : FromWorkspace  Tag=STV FromWs  VariableName=tuvar  SampleTime=1
      SigBuilderData=|
      | common.afterFinalStr = 'Extrapolate'
      | common.sampleTime = '1'
      | dataSet.timeRange = [0 25]
      | dataSet.name = 'Sheet1'
      | sbobj.Name = 'Signal Builder'
      | sbobj.Groups.Name = 'Sheet1'
      | sbobj.Groups.Signals(1).Name = 'Front_left_CP'
      | sbobj.Groups.Signals(1).XData = [0 1 2 3 4 5 6 7 8 9 10 11 12 13 14 15 16 17 18 19 20 21 22 23 24 25]
      | sbobj.Groups.Signals(1).YData = [1 1 1 1 1 1 0 0 0 0 0 0 0 0 0 0 0 0 0 0 0 0 0 0 0 1]
      | sbobj.Groups.Signals(2).Name = 'Right_left_CP'
      | sbobj.Groups.Signals(2).XData = [0 1 2 3 4 5 6 7 8 9 10 11 12 13 14 15 16 17 18 19 20 21 22 23 24 25]
      | sbobj.Groups.Signals(2).YData = [0 1 0 1 1 1 1 0 0 0 0 0 0 0 0 0 0 0 0 0 0 0 0 0 0 1]
      | sbobj.Groups.Signals(3).Name = 'Right_right_CP'
      | sbobj.Groups.Signals(3).XData = [0 1 2 3 4 5 6 7 8 9 10 11 12 13 14 15 16 17 18 19 20 21 22 23 24 25]
      | sbobj.Groups.Signals(3).YData = [0 1 1 1 1 1 0 0 0 0 0 0 0 0 0 0 0 0 0 0 0 0 0 0 0 1]
      | sbobj.Groups.Signals(4).Name = 'Driver_control'
      | sbobj.Groups.Signals(4).XData = [0 1 2 3 4 5 6 7 8 9 10 11 12 13 14 15 16 17 18 19 20 21 22 23 24 25]
      | sbobj.Groups.Signals(4).YData = [0 0 0 1 0 1 0 1 0 0 1 0 1 0 0 0 1 1 1 0 0 1 1 0 0 1]
      | sbobj.Groups.Signals(5).Name = 'Front_left_DC'
      | sbobj.Groups.Signals(5).XData = [0 1 2 3 4 5 6 7 8 9 10 11 12 13 14 15 16 17 18 19 20 21 22 23 24 25]
      | sbobj.Groups.Signals(5).YData = [1 1 1 1 1 1 1 1 1 1 0 0 0 0 0 1 1 1 1 1 0 0 1 1 1 0]
      | sbobj.Groups.Signals(6).Name = 'rear_left_DC'
      | sbobj.Groups.Signals(6).XData = [0 1 2 3 4 5 6 7 8 9 10 11 12 13 14 15 16 17 18 19 20 21 22 23 24 25]
      | sbobj.Groups.Signals(6).YData = [1 1 1 1 1 1 1 1 1 1 1 1 0 0 1 0 0 1 0 0 0 0 1 1 1 0]
      | sbobj.Groups.Signals(7).Name = 'rear_right_DC'
      | sbobj.Groups.Signals(7).XData = [0 1 2 3 4 5 6 7 8 9 10 11 12 13 14 15 16 17 18 19 20 21 22 23 24 25]
      | sbobj.Groups.Signals(7).YData = [1 1 1 1 1 1 1 1 1 1 1 0 0 0 0 1 1 1 1 1 1 1 1 1 0 0]
      | sbobj.Groups.Signals(8).Name = 'oject_detection'
      | sbobj.Groups.Signals(8).XData = [0 1 2 3 4 5 6 7 8 9 10 11 12 13 14 15 16 17 18 19 20 21 22 23 24 25]
      | sbobj.Groups.Signals(8).YData = [0 1 0 0 0 0 0 0 0 0 0 0 0 0 0 0 0 0 0 0 0 0 0 0 1 0]
      | sbobj.Groups.Signals(9).Name = 'Lock_Unlock'
      | sbobj.Groups.Signals(9).XData = [0 1 2 3 4 5 6 7 8 9 10 11 12 13 14 15 16 17 18 19 20 21 22 23 24 25]
      | sbobj.Groups.Signals(9).YData = [0 0 1 1 1 1 1 1 1 1 1 0 0 0 0 0 0 0 0 0 0 0 0 0 0 0]
      | sbobj.Groups.Signals(10).Name = 'iginition'
      | sbobj.Groups.Signals(10).XData = [0 1 2 3 4 5 6 7 8 9 10 11 12 13 14 15 16 17 18 19 20 21 22 23 24 25]
      | sbobj.Groups.Signals(10).YData = [0 1 1 1 1 1 1 1 1 1 1 1 1 1 1 1 1 1 1 1 1 1 1 1 1 1]
      | sbobj.Groups.TimeRange = [0 25]
  Front_left_CP : Outport  Tag=STV Outport
  Right_left_CP : Outport  Tag=STV Outport  Port=2
  Right_right_CP : Outport  Tag=STV Outport  Port=3
  Driver_control : Outport  Tag=STV Outport  Port=4
  Front_left_DC : Outport  Tag=STV Outport  Port=5
  rear_left_DC : Outport  Tag=STV Outport  Port=6
  rear_right_DC : Outport  Tag=STV Outport  Port=7
  oject_detection : Outport  Tag=STV Outport  Port=8
  Lock_Unlock : Outport  Tag=STV Outport  Port=9
  iginition : Outport  Tag=STV Outport  Port=10
  wires:
  Demux/1 -> Front_left_CP/1
  FromWs/1 -> Demux/1
  Demux/2 -> Right_left_CP/1
  Demux/3 -> Right_right_CP/1
  Demux/4 -> Driver_control/1
  Demux/5 -> Front_left_DC/1
  Demux/6 -> rear_left_DC/1
  Demux/7 -> rear_right_DC/1
  Demux/8 -> oject_detection/1
  Demux/9 -> Lock_Unlock/1
  Demux/10 -> iginition/1

== system Automated_features1/INPUT/Wiper_INPUTS/Signal Builder ==
  Demux : Demux  Tag=STV Demux  Outputs=5
      settings: DisplayOption=none
  FromWs : FromWorkspace  Tag=STV FromWs  VariableName=tuvar
      SigBuilderData=|
      | common.afterFinalStr = 'Extrapolate'
      | common.sampleTime = 0
      | dataSet.timeRange = [0 10]
      | dataSet.name = 'Group 1'
      | sbobj.Groups.Name = 'Group 1'
      | sbobj.Groups.Signals(1).Name = 'FC_Modes'
      | sbobj.Groups.Signals(1).XData = [0 1 2 3 4 5 6 7 8 9 10 11 12 13 14 15 16 17 18 19 20 21 22 23 24 25 26 27 28 29 30 31 32 33 34 35 36 37 38 39 40 41 42 43]
      | sbobj.Groups.Signals(1).YData = [0 1 1 1 1 1 1 1 1 1 1 1 2 2 2 2 2 2 2 2 3 3 3 3 3 4 4 4 4 4 5 5 5 6 6 6 6 6 6 6 6 6 6 6]
      | sbobj.Groups.Signals(2).Name = 'FC_ManualInput'
      | sbobj.Groups.Signals(2).XData = [0 1 2 3 4 5 6 7 8 9 10 11 12 13 14 15 16 17 18 19 20 21 22 23 24 25 26 27 28 29 30 31 32 33 34 35 36 37 38 39 40 41 42 43]
      | sbobj.Groups.Signals(2).YData = [0 0 0 0 0 0 0 0 0 0 0 0 0 0 0 0 0 0 0 0 0 0 0 0 0 0 0 0 0 0 0 0 0 0 15 20 36 50 65 69 80 85 90 98]
      | sbobj.Groups.Signals(3).Name = 'WC_BackS'
      | sbobj.Groups.Signals(3).XData = [0 1 2 3 4 5 6 7 8 9 10 11 12 13 14 15 16 17 18 19 20 21 22 23 24 25 26 27 28 29 30 31 32 33 34 35 36 37 38 39 40 41 42 43]
      | sbobj.Groups.Signals(3).YData = [0 1 1 1 1 1 1 1 1 1 1 1 0 0 0 0 0 0 0 0 0 0 0 0 0 0 0 0 0 0 0 0 0 0 0 0 0 0 0 0 0 0 0 0]
      | sbobj.Groups.Signals(4).Name = 'WC_Fronts'
      | sbobj.Groups.Signals(4).XData = [0 1 2 3 4 5 6 7 8 9 10 11 12 13 14 15 16 17 18 19 20 21 22 23 24 25 26 27 28 29 30 31 32 33 34 35 36 37 38 39 40 41 42 43]
      | sbobj.Groups.Signals(4).YData = [0 1 1 1 1 1 1 1 1 1 1 1 1 1 1 1 1 1 1 1 1 1 1 1 1 1 1 1 1 1 1 1 1 1 1 1 1 1 1 1 1 1 1 1]
      | sbobj.Groups.Signals(5).Name = 'WC_Status'
      | sbobj.Groups.Signals(5).XData = [0 1 2 3 4 5 6 7 8 9 10 11 12 13 14 15 16 17 18 19 20 21 22 23 24 25 26 27 28 29 30 31 32 33 34 35 36 37 38 39 40 41 42 43]
      | sbobj.Groups.Signals(5).YData = [0 1 1 1 1 1 1 1 1 1 1 1 1 1 1 1 1 1 1 1 1 1 1 1 1 1 1 1 1 1 1 1 1 1 1 1 1 1 1 1 1 1 1 1]
  FC_Modes : Outport  Tag=STV Outport
  FC_ManualInput : Outport  Tag=STV Outport  Port=2
  WC_BackS : Outport  Tag=STV Outport  Port=3
  WC_Fronts : Outport  Tag=STV Outport  Port=4
  WC_Status : Outport  Tag=STV Outport  Port=5
  wires:
  FromWs/1 -> Demux/1
  Demux/1 -> FC_Modes/1
  Demux/2 -> FC_ManualInput/1
  Demux/3 -> WC_BackS/1
  Demux/4 -> WC_Fronts/1
  Demux/5 -> WC_Status/1

== system Automated_features1/MODULES/	POWER_WINDOW/Subsystem4 ==
  Ig_sw : Inport
  object : Inport  Port=2
  Front_left_subsystem : Subsystem
  Rear_right_Subsystem : Subsystem
  driver_control_Subsystem : Subsystem
  rear_left_Subsystem : Subsystem
  Out_warn : Outport
  Out_FL : Outport  Port=2
  Out_RL_warn : Outport  Port=3
  Out_RL : Outport  Port=4
  Out_RR_warn : Outport  Port=5
  Out_RR : Outport  Port=6
  Out_DC_warn : Outport  Port=7
  Out_DC : Outport  Port=8
  wires:
  [lock_unlock_button] -> rear_left_Subsystem/1(lock/unlock), Rear_right_Subsystem/1(lock/unlock), Front_left_subsystem/1(lock/unlock)  "lock/unlock"
  Ig_sw/1 -> Rear_right_Subsystem/Enable, rear_left_Subsystem/Enable, driver_control_Subsystem/Enable, Front_left_subsystem/Enable
  object/1 -> Front_left_subsystem/4(object), driver_control_Subsystem/2(object), Rear_right_Subsystem/4(object), rear_left_Subsystem/4(object)  "object"
  Front_left_subsystem/2(Outport1) -> Out_FL/1
  Front_left_subsystem/1(Outport) -> Out_warn/1
  rear_left_Subsystem/2(Outport1) -> Out_RL/1
  rear_left_Subsystem/1(Outport) -> Out_RL_warn/1
  Rear_right_Subsystem/2(Outport1) -> Out_RR/1
  Rear_right_Subsystem/1(Outport) -> Out_RR_warn/1
  driver_control_Subsystem/2(Outport1) -> Out_DC/1
  driver_control_Subsystem/1(Outport) -> Out_DC_warn/1
  [Front_left_button_CP] -> Front_left_subsystem/2(In_fl_b)
  [Front_left_button_driver_side] -> Front_left_subsystem/3(In_fl_Dc)
  [rear_left_button_CP] -> rear_left_Subsystem/2(In2)
  [rear_left_button_driver_side] -> rear_left_Subsystem/3(In3)
  [rear_right_button_CP] -> Rear_right_Subsystem/2(In2)
  [rear_right_button_driver_side] -> Rear_right_Subsystem/3(In3)
  [driver_switch] -> driver_control_Subsystem/1(In1)

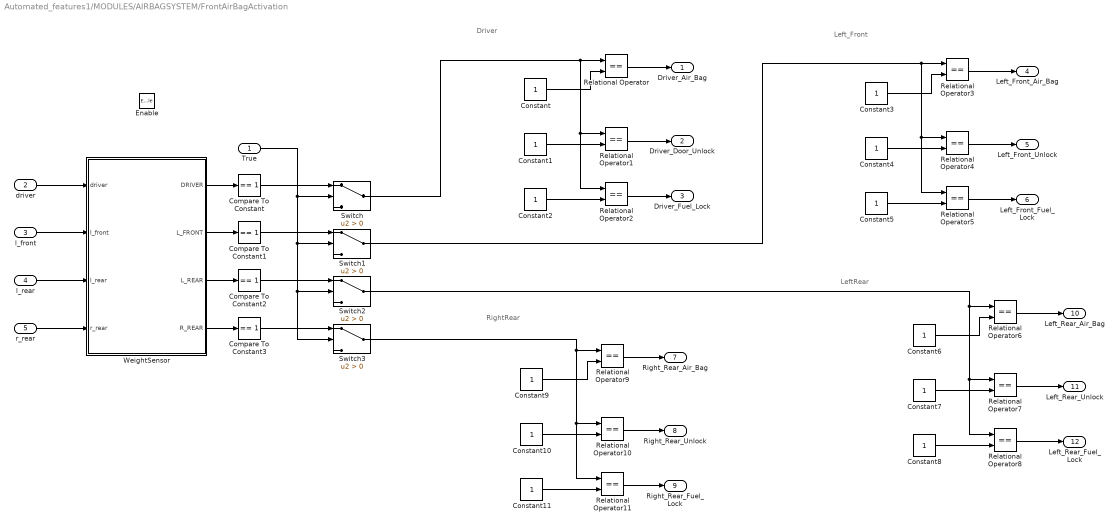
== system Automated_features1/MODULES/AIRBAGSYSTEM/FrontAirBagActivation ==
  note: RightRear
  note: LeftRear
  note: Left_Front
  note: Driver
  True : Inport
  driver : Inport  Port=2
  l_front : Inport  Port=3
  l_rear : Inport  Port=4
  r_rear : Inport  Port=5
  Enable : EnablePort
  Compare To Constant{,1..3} (4 alike) : simulink/Logic and Bit Operations/Compare To Constant  relop===  const=1  OutDataTypeStr=boolean
  Constant{,1..11} (12 alike) : Constant
  Relational Operator{,1..11} (12 alike) : RelationalOperator  Operator===  OutDataTypeStr=boolean  RndMeth=Simplest
  Switch{,1..3} (4 alike) : Switch  Criteria=u2 > Threshold
  WeightSensor : MATLAB Function  TreatAsAtomicUnit=on
  Driver_Air_Bag : Outport
  Driver_Door_Unlock : Outport  Port=2
  Driver_Fuel_Lock : Outport  Port=3
  Left_Front_Air_Bag : Outport  Port=4
  Left_Front_Unlock : Outport  Port=5
  Left_Front_Fuel_Lock : Outport  Port=6
  Right_Rear_Air_Bag : Outport  Port=7
  Right_Rear_Unlock : Outport  Port=8
  Right_Rear_Fuel_Lock : Outport  Port=9
  Left_Rear_Air_Bag : Outport  Port=10
  Left_Rear_Unlock : Outport  Port=11
  Left_Rear_Fuel_Lock : Outport  Port=12
  wires:
  WeightSensor/2(L_FRONT) -> Compare To Constant1/1
  WeightSensor/1(DRIVER) -> Compare To Constant/1
  WeightSensor/3(L_REAR) -> Compare To Constant2/1
  WeightSensor/4(R_REAR) -> Compare To Constant3/1
  True/1 -> Switch3/2, Switch2/2, Switch1/2, Switch/2
  Compare To Constant/1 -> Switch/1
  Compare To Constant1/1 -> Switch1/1
  Compare To Constant2/1 -> Switch2/1
  Compare To Constant3/1 -> Switch3/1
  Constant2/1 -> Relational Operator2/2
  Switch/1 -> Relational Operator2/1, Relational Operator1/1, Relational Operator/1
  Constant1/1 -> Relational Operator1/2
  Constant/1 -> Relational Operator/2
  Constant4/1 -> Relational Operator4/2
  Constant5/1 -> Relational Operator5/2
  Switch1/1 -> Relational Operator5/1, Relational Operator4/1, Relational Operator3/1
  Constant3/1 -> Relational Operator3/2
  Constant7/1 -> Relational Operator7/2
  Constant6/1 -> Relational Operator6/2
  Switch2/1 -> Relational Operator8/1, Relational Operator7/1, Relational Operator6/1
  Constant8/1 -> Relational Operator8/2
  Switch3/1 -> Relational Operator11/1, Relational Operator10/1, Relational Operator9/1
  Constant11/1 -> Relational Operator11/2
  Constant10/1 -> Relational Operator10/2
  Constant9/1 -> Relational Operator9/2
  driver/1 -> WeightSensor/1(driver)
  l_front/1 -> WeightSensor/2(l_front)
  l_rear/1 -> WeightSensor/3(l_rear)
  r_rear/1 -> WeightSensor/4(r_rear)
  Relational Operator3/1 -> Left_Front_Air_Bag/1
  Relational Operator4/1 -> Left_Front_Unlock/1
  Relational Operator5/1 -> Left_Front_Fuel_Lock/1
  Relational Operator9/1 -> Right_Rear_Air_Bag/1
  Relational Operator10/1 -> Right_Rear_Unlock/1
  Relational Operator11/1 -> Right_Rear_Fuel_Lock/1
  Relational Operator6/1 -> Left_Rear_Air_Bag/1
  Relational Operator7/1 -> Left_Rear_Unlock/1
  Relational Operator8/1 -> Left_Rear_Fuel_Lock/1
  Relational Operator/1 -> Driver_Air_Bag/1
  Relational Operator1/1 -> Driver_Door_Unlock/1
  Relational Operator2/1 -> Driver_Fuel_Lock/1

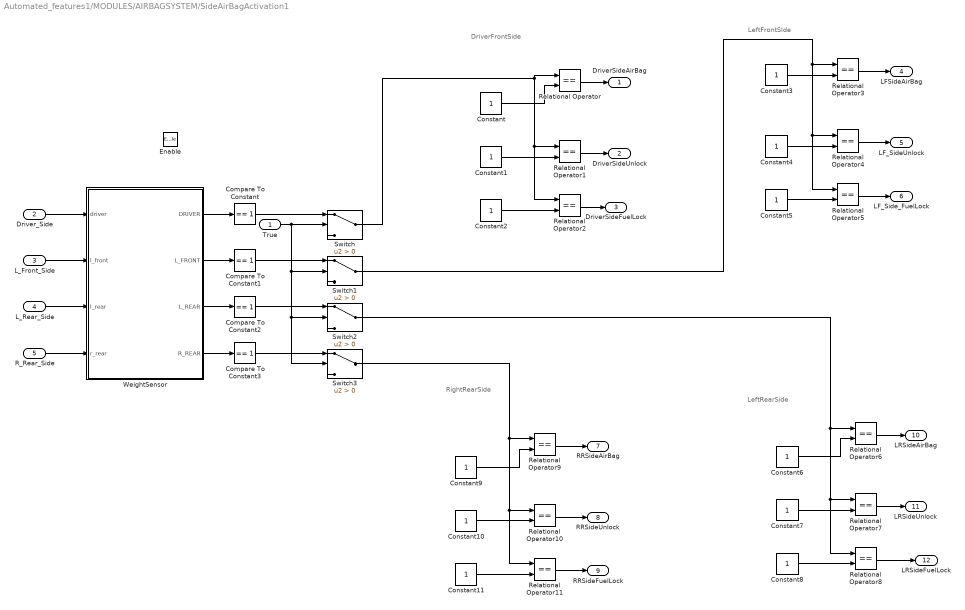
== system Automated_features1/MODULES/AIRBAGSYSTEM/SideAirBagActivation1 ==
  note: RightRearSide
  note: LeftRearSide
  note: LeftFrontSIde
  note: DriverFrontSide
  True : Inport
  Driver_Side : Inport  Port=2
  L_Front_Side : Inport  Port=3
  L_Rear_Side : Inport  Port=4
  R_Rear_Side : Inport  Port=5
  Enable : EnablePort
  Compare To Constant{,1..3} (4 alike) : simulink/Logic and Bit Operations/Compare To Constant  relop===  const=1  OutDataTypeStr=boolean
  Constant{,1..11} (12 alike) : Constant
  Relational Operator{,1..11} (12 alike) : RelationalOperator  Operator===  OutDataTypeStr=boolean  RndMeth=Simplest
  Switch{,1..3} (4 alike) : Switch  Criteria=u2 > Threshold
  WeightSensor : MATLAB Function  TreatAsAtomicUnit=on
  DriverSideAirBag : Outport
  DriverSideUnlock : Outport  Port=2
  DriverSideFuelLock : Outport  Port=3
  LFSideAirBag : Outport  Port=4
  LF_SideUnlock : Outport  Port=5
  LF_Side_FuelLock : Outport  Port=6
  RRSideAirBag : Outport  Port=7
  RRSideUnlock : Outport  Port=8
  RRSideFuelLock : Outport  Port=9
  LRSideAirBag : Outport  Port=10
  LRSideUnlock : Outport  Port=11
  LRSideFuelLock : Outport  Port=12
  wires:
  WeightSensor/2(L_FRONT) -> Compare To Constant1/1
  WeightSensor/3(L_REAR) -> Compare To Constant2/1
  WeightSensor/4(R_REAR) -> Compare To Constant3/1
  Compare To Constant1/1 -> Switch1/1
  True/1 -> Switch3/2, Switch2/2, Switch1/2, Switch/2
  WeightSensor/1(DRIVER) -> Compare To Constant/1
  Compare To Constant3/1 -> Switch3/1
  Compare To Constant2/1 -> Switch2/1
  Compare To Constant/1 -> Switch/1
  Driver_Side/1 -> WeightSensor/1(driver)
  R_Rear_Side/1 -> WeightSensor/4(r_rear)
  L_Rear_Side/1 -> WeightSensor/3(l_rear)
  L_Front_Side/1 -> WeightSensor/2(l_front)
  Constant2/1 -> Relational Operator2/2
  Constant1/1 -> Relational Operator1/2
  Constant/1 -> Relational Operator/2
  Switch/1 -> Relational Operator2/1, Relational Operator1/1, Relational Operator/1
  Constant4/1 -> Relational Operator4/2
  Constant3/1 -> Relational Operator3/2
  Constant5/1 -> Relational Operator5/2
  Switch1/1 -> Relational Operator5/1, Relational Operator4/1, Relational Operator3/1
  Constant8/1 -> Relational Operator8/2
  Switch2/1 -> Relational Operator8/1, Relational Operator7/1, Relational Operator6/1
  Constant7/1 -> Relational Operator7/2
  Constant6/1 -> Relational Operator6/2
  Constant11/1 -> Relational Operator11/2
  Switch3/1 -> Relational Operator11/1, Relational Operator10/1, Relational Operator9/1
  Constant9/1 -> Relational Operator9/2
  Constant10/1 -> Relational Operator10/2
  Relational Operator/1 -> DriverSideAirBag/1
  Relational Operator1/1 -> DriverSideUnlock/1
  Relational Operator2/1 -> DriverSideFuelLock/1
  Relational Operator3/1 -> LFSideAirBag/1
  Relational Operator4/1 -> LF_SideUnlock/1
  Relational Operator5/1 -> LF_Side_FuelLock/1
  Relational Operator9/1 -> RRSideAirBag/1
  Relational Operator10/1 -> RRSideUnlock/1
  Relational Operator11/1 -> RRSideFuelLock/1
  Relational Operator6/1 -> LRSideAirBag/1
  Relational Operator7/1 -> LRSideUnlock/1
  Relational Operator8/1 -> LRSideFuelLock/1

== system Automated_features1/MODULES/ALARM_SYSTEM/Main_Alarm ==
  data2 : Inport
  AND : Logic  Inputs=3  IconShape=distinctive  AllPortsSameDT=off  OutDataTypeStr=boolean
  AND1 : Logic  Inputs=3  IconShape=distinctive  AllPortsSameDT=off  OutDataTypeStr=boolean
  AND2 : Logic  IconShape=distinctive  AllPortsSameDT=off  OutDataTypeStr=boolean
  AND3 : Logic  IconShape=distinctive  AllPortsSameDT=off  OutDataTypeStr=boolean
  ARMED : Stateflow chart  TreatAsAtomicUnit=on
  Compare To Constant : simulink/Logic and Bit Operations/Compare To Constant  relop===  const=0  OutDataTypeStr=boolean
  Compare To Constant2 : simulink/Logic and Bit Operations/Compare To Constant  relop===  const=1  OutDataTypeStr=boolean
  Compare To Constant3 : simulink/Logic and Bit Operations/Compare To Constant  relop===  const=1  OutDataTypeStr=boolean
  Compare To Zero : simulink/Logic and Bit Operations/Compare To Zero  relop===  OutDataTypeStr=boolean
  Compare To Zero1 : simulink/Logic and Bit Operations/Compare To Zero  relop===  OutDataTypeStr=boolean
  Display3 : DisplayBlock  LabelPosition=Hide  Format=short  Transparency=1
  Display4 : DisplayBlock  LabelPosition=Hide  Format=short  Transparency=1
  Lamp : LampBlock
  Pre_Alarm : Stateflow chart  TreatAsAtomicUnit=on
  Rotary Switch : RotarySwitchBlock
      settings: Values={{'zero', 'one', 'Unlocking'}, [0 1 2]}
  String Constant : StringConstant  String="\"DISARMED!\""
  String Constant2 : StringConstant  String="\"Horn And Lights are ON!\""
  Switch : Switch  Criteria=u2 ~= 0
  Switch1 : Switch  Criteria=u2 ~= 0
  Toggle Switch : ToggleSwitchBlock
      settings: Values={{'Off', 'On'}, [0 1]}
  tag scope: Alarm_ARMED=global, Disarmed=global, Prealarm_ARMED=global
  wires:
  [Ignition] -> Compare To Constant2/1, AND/1
  AND/1 -> Compare To Constant/1
  [CAR_ON] -> AND/2
  ARMED/1(data1) -> AND1/3, Compare To Constant3/1
  data2/1 -> Compare To Zero1/1, AND/3
  Compare To Constant2/1 -> AND1/1
  [RKE] -> AND1/2, Compare To Zero/1, AND2/2  "RKE"
  AND1/1 -> Switch/2
  String Constant/1 -> Switch/1
  Switch/1 -> [Disarmed]
  Pre_Alarm/1(data1) -> Switch1/2
  String Constant2/1 -> Switch1/1
  Compare To Constant/1 -> AND2/1
  Compare To Constant3/1 -> [Alarm_ARMED]
  AND2/1 -> ARMED/1(data)
  Compare To Zero/1 -> AND3/1
  AND3/1 -> Pre_Alarm/1(data)
  Compare To Zero1/1 -> AND3/2
  Switch1/1 -> [Prealarm_ARMED]

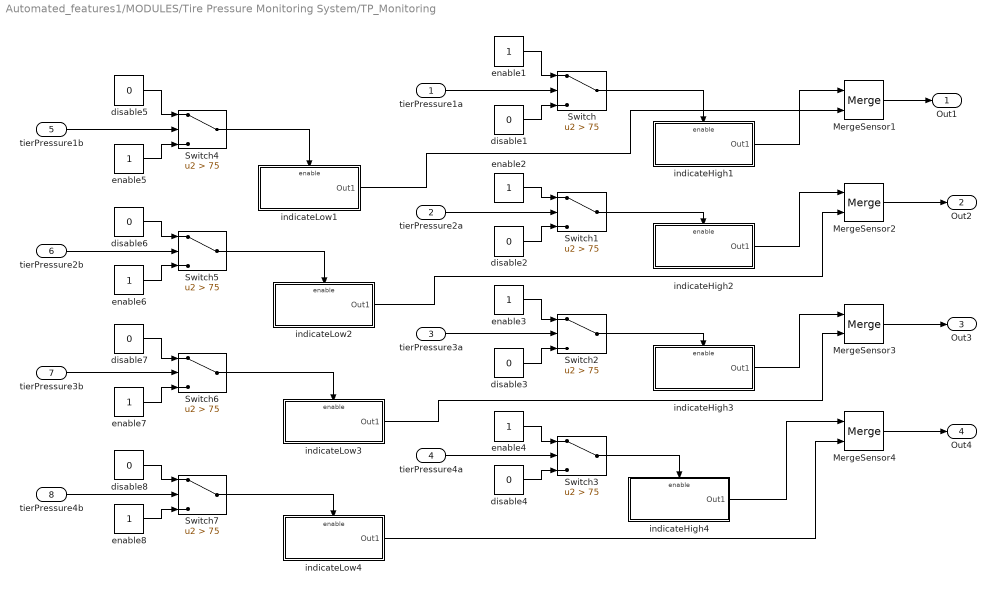
== system Automated_features1/MODULES/Tire Pressure Monitoring System/TP_Monitoring ==
  tierPressure1a : Inport
  tierPressure2a : Inport  Port=2
  tierPressure3a : Inport  Port=3
  tierPressure4a : Inport  Port=4
  tierPressure1b : Inport  Port=5
  tierPressure2b : Inport  Port=6
  tierPressure3b : Inport  Port=7
  tierPressure4b : Inport  Port=8
  MergeSensor{1..4} (4 alike) : Merge
  Switch{,1..7} (8 alike) : Switch  Criteria=u2 > Threshold  Threshold=75
  disable{1..8} (8 alike) : Constant  Value=0
  enable{1..8} (8 alike) : Constant
  indicateHigh1 : Subsystem  TreatAsAtomicUnit=on
  indicateHigh2 : Subsystem  TreatAsAtomicUnit=on
  indicateHigh3 : Subsystem  TreatAsAtomicUnit=on
  indicateHigh4 : Subsystem  TreatAsAtomicUnit=on
  indicateLow1 : Subsystem  TreatAsAtomicUnit=on
  indicateLow2 : Subsystem  TreatAsAtomicUnit=on
  indicateLow3 : Subsystem  TreatAsAtomicUnit=on
  indicateLow4 : Subsystem  TreatAsAtomicUnit=on
  Out1 : Outport
  Out2 : Outport  Port=2
  Out3 : Outport  Port=3
  Out4 : Outport  Port=4
  wires:
  enable1/1 -> Switch/1
  tierPressure3a/1 -> Switch2/2
  disable1/1 -> Switch/3
  disable3/1 -> Switch2/3
  enable2/1 -> Switch1/1
  tierPressure1a/1 -> Switch/2
  disable4/1 -> Switch3/3
  disable2/1 -> Switch1/3
  enable4/1 -> Switch3/1
  tierPressure2a/1 -> Switch1/2
  tierPressure4a/1 -> Switch3/2
  enable3/1 -> Switch2/1
  disable8/1 -> Switch7/1
  enable8/1 -> Switch7/3
  disable6/1 -> Switch5/1
  enable6/1 -> Switch5/3
  enable7/1 -> Switch6/3
  enable5/1 -> Switch4/3
  disable5/1 -> Switch4/1
  tierPressure2b/1 -> Switch5/2
  tierPressure3b/1 -> Switch6/2
  tierPressure1b/1 -> Switch4/2
  disable7/1 -> Switch6/1
  tierPressure4b/1 -> Switch7/2
  MergeSensor1/1 -> Out1/1
  MergeSensor2/1 -> Out2/1
  MergeSensor3/1 -> Out3/1
  MergeSensor4/1 -> Out4/1
  Switch3/1 -> indicateHigh4/Enable
  Switch2/1 -> indicateHigh3/Enable
  Switch1/1 -> indicateHigh2/Enable
  Switch/1 -> indicateHigh1/Enable
  Switch7/1 -> indicateLow4/Enable
  Switch6/1 -> indicateLow3/Enable
  Switch5/1 -> indicateLow2/Enable
  Switch4/1 -> indicateLow1/Enable
  indicateHigh1/1(Out1) -> MergeSensor1/1
  indicateLow1/1(Out1) -> MergeSensor1/2
  indicateHigh2/1(Out1) -> MergeSensor2/1
  indicateLow2/1(Out1) -> MergeSensor2/2
  indicateHigh3/1(Out1) -> MergeSensor3/1
  indicateLow3/1(Out1) -> MergeSensor3/2
  indicateHigh4/1(Out1) -> MergeSensor4/1
  indicateLow4/1(Out1) -> MergeSensor4/2

== system Automated_features1/MODULES/WIPER_CONTROL/Atomic Subsystem ==
  Inport : Inport
  Clock : Clock
      settings: Decimation=5
  Compare To Constant : simulink/Logic and Bit Operations/Compare To Constant  relop===  const=1  OutDataTypeStr=boolean
  Compare To Constant5 : simulink/Logic and Bit Operations/Compare To Constant  relop===  const=1  OutDataTypeStr=boolean
  Gain : Gain  Gain=10
  Relational Operator : RelationalOperator  Operator=<  OutDataTypeStr=boolean  RndMeth=Simplest
  tag scope: BW_Display=global
  wires:
  Compare To Constant5/1 -> [BW_Display]
  Inport/1 -> Compare To Constant/1
  Gain/1 -> Relational Operator/2
  Clock/1 -> Relational Operator/1
  Relational Operator/1 -> Compare To Constant5/1
  Compare To Constant/1 -> Gain/1

== system Automated_features1/MODULES/WIPER_CONTROL/Atomic Subsystem1 ==
  Inport : Inport
  Auto_Modes : Subsystem
  Display : Display
  Manual_mode : Subsystem
  wires:
  [FW_Modes] -> Manual_mode/1(In1), Auto_Modes/1(In1)
  Inport/1 -> Display/1
